simulink model "task3-Simulink"  (R2015b)
settings: Solver=ode15s  StartTime=0.0  StopTime=3  RelTol=1e-3
values from neighbouring files (symbols this model uses):
  J = 60*10^-7    (= 6e-06)    [All Tasks Compiled.m]
  Kd = Cv*n0/5    (= 0.00143)    [All Tasks Compiled.m]
  Kemf = 4.555*10^(-3)*60/(2*pi)    (= 0.043497045947)    [All Tasks Compiled.m]
  Km = 43.5*10^-3    (= 0.0435)    [All Tasks Compiled.m]
  Kp = 2    [All Tasks Compiled.m]
  L = 0.1    [All Tasks Compiled.m]
  R = 1.45    [All Tasks Compiled.m]
settings Model: Creator=atang  LastModifiedBy=daniella.a
settings DataIOCC: LimitDataPoints=off

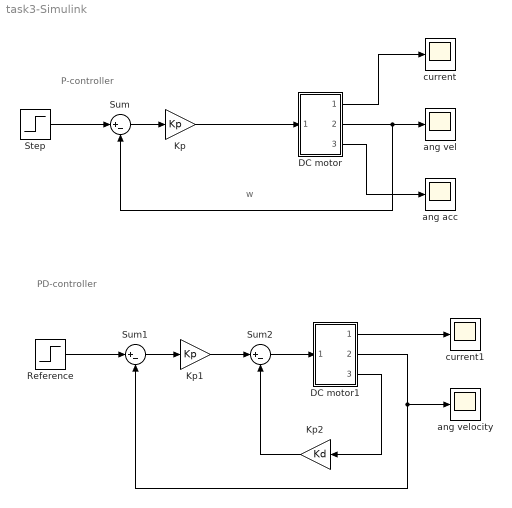
== system task3-Simulink ==
  note: PD-controller
  note: P-controller
  note: w
  DC motor : Subsystem
  DC motor1 : Subsystem
  Kp : Gain  Gain=Kp
  Kp1 : Gain  Gain=Kp
  Kp2 : Gain  Gain=Kd
  "Reference " : Step  After=12  SampleTime=0
  Step : Step  After=12  SampleTime=0
  Sum : Sum  Inputs=|+-
  Sum1 : Sum  Inputs=|+-
  Sum2 : Sum  Inputs=|+-
  ang acc : Scope
  "ang vel " : Scope
  "ang velocity " : Scope
  current : Scope
  current1 : Scope
  wires:
  DC motor/1(Out1) -> current/1
  DC motor/2(Out2) -> Sum/2, "ang vel "/1
  Step/1 -> Sum/1
  Sum/1 -> Kp/1
  Kp/1 -> DC motor/1(In1)
  DC motor/3(Out3) -> ang acc/1
  DC motor1/1(Out1) -> current1/1
  DC motor1/2(Out2) -> "ang velocity "/1, Sum1/2
  "Reference "/1 -> Sum1/1
  Sum1/1 -> Kp1/1
  DC motor1/3(Out3) -> Kp2/1
  Kp1/1 -> Sum2/1
  Kp2/1 -> Sum2/2
  Sum2/1 -> DC motor1/1(In1)

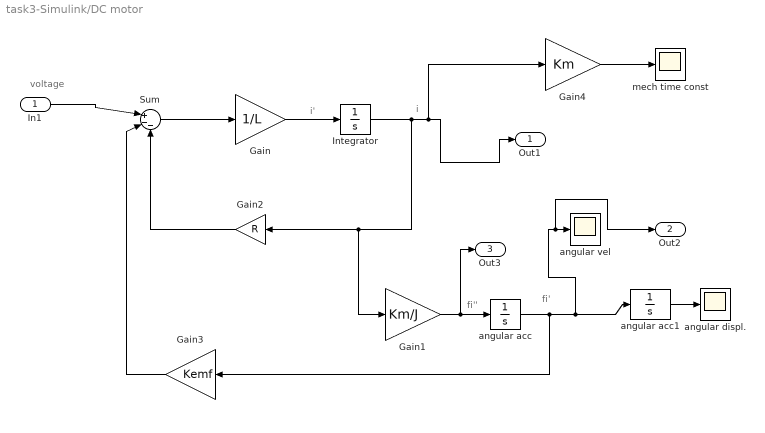
== system task3-Simulink/DC motor ==
  note: voltage
  note: fi'
  note: fi''
  note: i
  note: i'
  In1 : Inport
  Gain : Gain  Gain=1/L
  Gain1 : Gain  Gain=Km/J
  Gain2 : Gain  Gain=R
  Gain3 : Gain  Gain=Kemf
  Gain4 : Gain  Gain=Km
  Integrator : Integrator
  Sum : Sum  Inputs=|+--
  angular acc : Integrator
  angular acc1 : Integrator
  angular displ. : Scope
  angular vel : Scope
  mech time const : Scope
  Out1 : Outport
  Out2 : Outport  Port=2
  Out3 : Outport  Port=3
  wires:
  Sum/1 -> Gain/1
  Gain/1 -> Integrator/1
  Integrator/1 -> Gain1/1, Gain2/1, Gain4/1, Out1/1
  Gain2/1 -> Sum/3
  Gain1/1 -> Out3/1, angular acc/1
  angular acc/1 -> Gain3/1, Out2/1, angular vel/1, angular acc1/1
  Gain3/1 -> Sum/2
  angular acc1/1 -> angular displ./1
  Gain4/1 -> mech time const/1
  In1/1 -> Sum/1

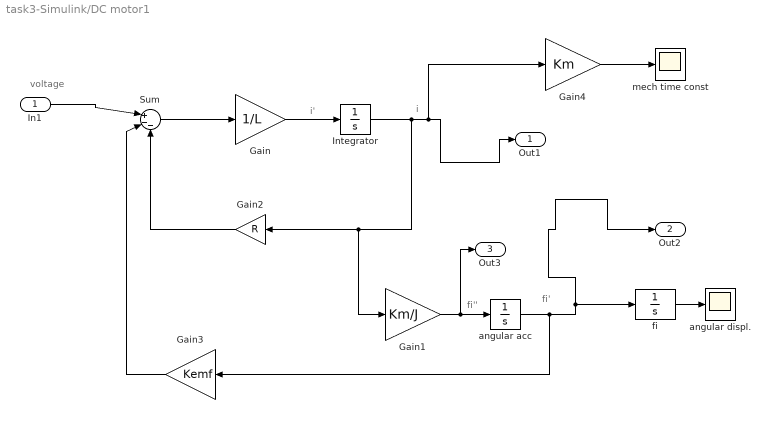
== system task3-Simulink/DC motor1 ==
  note: i'
  note: i
  note: fi''
  note: fi'
  note: voltage
  In1 : Inport
  Gain : Gain  Gain=1/L
  Gain1 : Gain  Gain=Km/J
  Gain2 : Gain  Gain=R
  Gain3 : Gain  Gain=Kemf
  Gain4 : Gain  Gain=Km
  Integrator : Integrator
  Sum : Sum  Inputs=|+--
  angular acc : Integrator
  angular displ. : Scope
  fi : Integrator
  mech time const : Scope
  Out1 : Outport
  Out2 : Outport  Port=2
  Out3 : Outport  Port=3
  wires:
  In1/1 -> Sum/1
  Gain4/1 -> mech time const/1
  fi/1 -> angular displ./1
  Gain3/1 -> Sum/2
  angular acc/1 -> fi/1, Out2/1, Gain3/1
  Gain1/1 -> angular acc/1, Out3/1
  Gain2/1 -> Sum/3
  Integrator/1 -> Out1/1, Gain4/1, Gain2/1, Gain1/1
  Gain/1 -> Integrator/1
  Sum/1 -> Gain/1
